simulink model "position_force"  (R2021a)
settings: Solver=FixedStepAuto  StartTime=0.0  StopTime=5  FixedStep=0.001  RelTol=1e-3
values from neighbouring files (symbols this model uses):
  k_fi = 2*eye(3)    [params.m]
  k_fp = 10*eye(3)    [params.m]
  kd = 2*z*w    [params.m]
  kp = w^2    [params.m]
  Md = 0.035*diag([1 1 1])    [params.m]
settings Model: Creator=Sebastiano  LastModifiedBy=antoninoparisi
settings SolverCC: AlgebraicLoopSolver=TrustRegion
settings DebuggingCC: SFMachineParentedDataDiag=warning

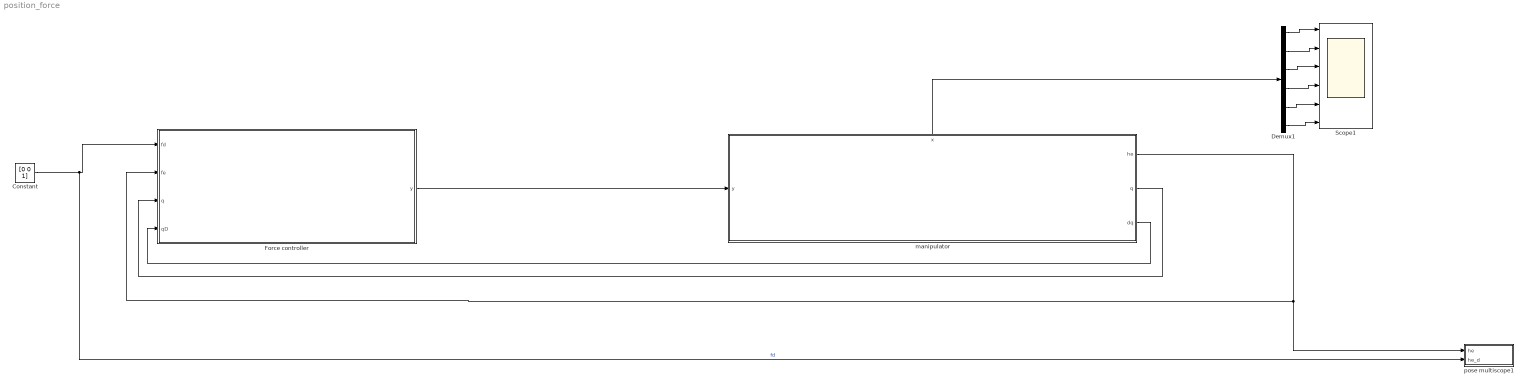
== system position_force ==
  Constant : Constant  Value=[0 0 1]  VectorParams1D=off  SampleTime=0.001
  Demux1 : Demux  Outputs=6
  Force controller : Subsystem
  Scope1 : Scope  NumInputPorts=6
  manipulator : Subsystem
      settings: PortSchema="{\"entries\":[{\"content\":{\"sides\":[{\"content\":{\"connectorIds\":[\"In1\"]},\"type\":\"ConnectorPlacement.EquallySpacedRectSide\",\"uuid\":\"0aa94650-4609-4b6c-9a82-adf30db4dc8c\"},{\"content\":{\"connectorIds\":[\"Out1\",\"Out2\",\"Out3\"],\"side\":\"RIGHT\"},\"type\":\"ConnectorPlacement.EquallySpacedRectSide\",\"uuid\":\"eb872eea-8278-41dd-b116-0828b4bf12ba\"},{\"content\":{\"connectorIds\":[\"Out4\"],\"side\":\"TOP\"},\"type\":\"ConnectorPlacement.EquallySpacedRectSide\",\"uuid\":\"ce640c9d-a400-4b3a-8367-eeadb4eb804b\"}]},\"type\":\"ConnectorPlacement.EquallySpacedConnector\",\"uuid\":\"b8e51044-d9d2-481c-9adb-6cf6a7f6c61e\"}],\"packageUris\":[\"http://schema.mathworks.com/mf0/Connector/R2020b\"],\"version\":\"1.0\"}"
  pose multiscope1 : Subsystem
  wires:
  Constant/1 -> pose multiscope1/2(he_d), Force controller/1(fd)  "fd"
  manipulator/2(q) -> Force controller/3(q)
  manipulator/3(dq) -> Force controller/4(qD)
  manipulator/1(he) -> pose multiscope1/1(he), Force controller/2(fe)
  manipulator/4(x) -> Demux1/1
  Demux1/1 -> Scope1/1
  Demux1/4 -> Scope1/4
  Demux1/5 -> Scope1/5
  Demux1/3 -> Scope1/3
  Demux1/6 -> Scope1/6
  Demux1/2 -> Scope1/2
  Force controller/1(y) -> manipulator/1(y)

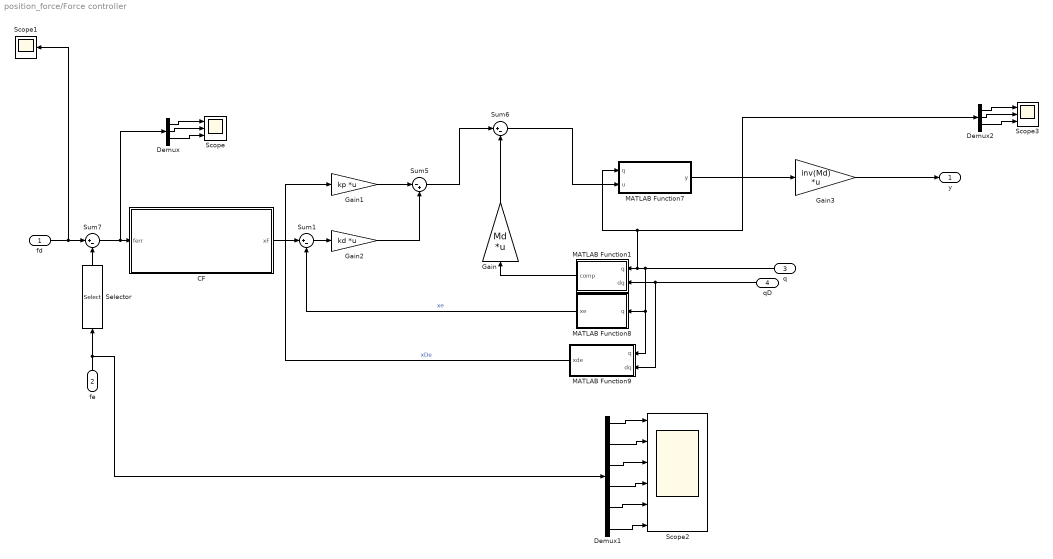
== system position_force/Force controller ==
  fd : Inport
  fe : Inport  Port=2
  q : Inport  Port=3
  qD : Inport  Port=4
  CF : Subsystem
  Demux : Demux  Outputs=3
  Demux1 : Demux  Outputs=6
  Demux2 : Demux  Outputs=3
  Gain : Gain  Gain=Md  Multiplication=Matrix(K*u) (u vector)
  Gain1 : Gain  Gain=kp  Multiplication=Matrix(K*u) (u vector)
  Gain2 : Gain  Gain=kd  Multiplication=Matrix(K*u) (u vector)
  Gain3 : Gain  Gain=inv(Md)  Multiplication=Matrix(K*u) (u vector)
  MATLAB Function1 : MATLAB Function  TreatAsAtomicUnit=on
  MATLAB Function7 : MATLAB Function  TreatAsAtomicUnit=on
  MATLAB Function8 : MATLAB Function  TreatAsAtomicUnit=on
  MATLAB Function9 : MATLAB Function  TreatAsAtomicUnit=on
  Scope : Scope  NumInputPorts=3
  Scope1 : Scope
  Scope2 : Scope  NumInputPorts=6
  Scope3 : Scope  NumInputPorts=3
  Selector : Selector  InputPortWidth=6  IndexOptions=Starting index (dialog)  Indices=1  OutputSizes=3
  Sum1 : Sum  Inputs=|+-
  Sum5 : Sum  Inputs=|-+
  Sum6 : Sum  Inputs=|+-
  Sum7 : Sum  Inputs=|+-
  y : Outport
  wires:
  fd/1 -> Scope1/1, Sum7/1
  Sum1/1 -> Gain2/1
  Sum5/1 -> Sum6/1
  MATLAB Function9/1(xde) -> Gain1/1  "xDe"
  Gain1/1 -> Sum5/1
  MATLAB Function1/1(comp) -> Gain/1
  Sum6/1 -> MATLAB Function7/2(u)
  Gain2/1 -> Sum5/2
  MATLAB Function8/1(xe) -> Sum1/2  "xe"
  Sum7/1 -> Demux/1, CF/1(ferr)
  CF/1(xF) -> Sum1/1
  qD/1 -> MATLAB Function9/2(dq), MATLAB Function1/2(dq)
  q/1 -> Demux2/1, MATLAB Function7/1(q), MATLAB Function1/1(q), MATLAB Function9/1(q), MATLAB Function8/1(q)
  Demux/1 -> Scope/1
  Demux/2 -> Scope/2
  Demux/3 -> Scope/3
  Gain/1 -> Sum6/2
  MATLAB Function7/1(y) -> Gain3/1
  Selector/1 -> Sum7/2
  Demux1/1 -> Scope2/1
  fe/1 -> Demux1/1, Selector/1
  Demux1/2 -> Scope2/2
  Demux1/4 -> Scope2/4
  Demux1/6 -> Scope2/6
  Demux1/5 -> Scope2/5
  Demux1/3 -> Scope2/3
  Demux2/3 -> Scope3/3
  Demux2/2 -> Scope3/2
  Gain3/1 -> y/1
  Demux2/1 -> Scope3/1

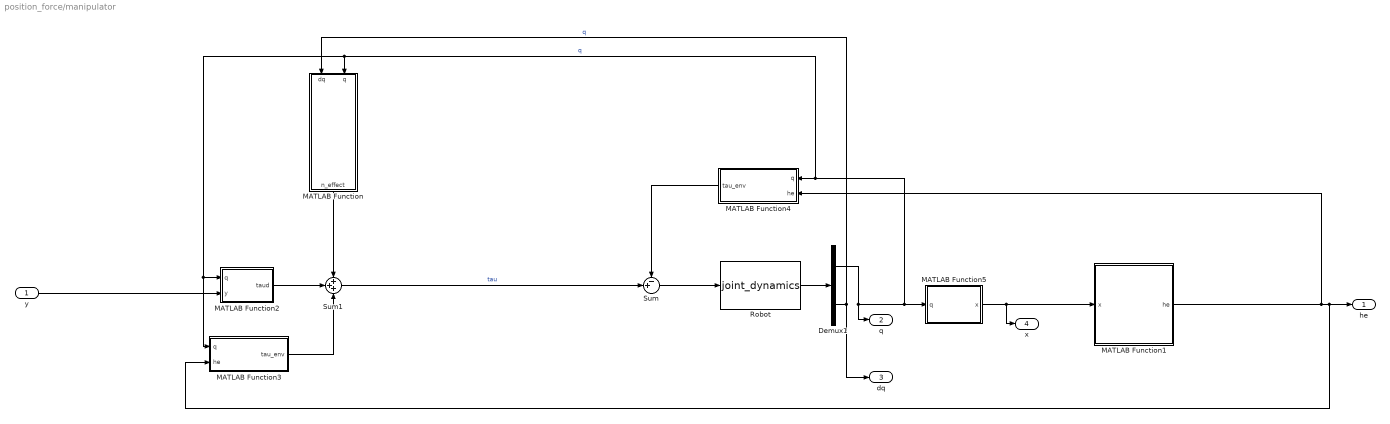
== system position_force/manipulator ==
  y : Inport
  Demux1 : Demux  Outputs=[3, 3]
  MATLAB Function : MATLAB Function  TreatAsAtomicUnit=on
  MATLAB Function1 : MATLAB Function  TreatAsAtomicUnit=on
  MATLAB Function2 : MATLAB Function  TreatAsAtomicUnit=on
  MATLAB Function3 : MATLAB Function  TreatAsAtomicUnit=on
  MATLAB Function4 : MATLAB Function  TreatAsAtomicUnit=on
  MATLAB Function5 : MATLAB Function  TreatAsAtomicUnit=on
  Robot : S-Function  FunctionName=joint_dynamics  Parameters=robot  SFunctionDeploymentMode=off  EnableBusSupport=off
  Sum : Sum  Inputs=-+|
  Sum1 : Sum  Inputs=+++
  he : Outport
  q : Outport  Port=2
  dq : Outport  Port=3
  x : Outport  Port=4
  wires:
  Sum/1 -> Robot/1
  Robot/1 -> Demux1/1
  MATLAB Function4/1(tau_env) -> Sum/1
  MATLAB Function5/1(x) -> x/1, MATLAB Function1/1(x)
  MATLAB Function1/1(he) -> MATLAB Function4/2(he), MATLAB Function3/2(he), he/1
  Demux1/1 -> MATLAB Function5/1(q), MATLAB Function/2(q), MATLAB Function3/1(q), MATLAB Function2/1(q), MATLAB Function4/1(q), q/1  "q"
  y/1 -> MATLAB Function2/2(y)
  MATLAB Function/1(n_effect) -> Sum1/1
  Sum1/1 -> Sum/2  "tau"
  MATLAB Function3/1(tau_env) -> Sum1/3
  MATLAB Function2/1(taud) -> Sum1/2
  Demux1/2 -> dq/1, MATLAB Function/1(dq)  "q"

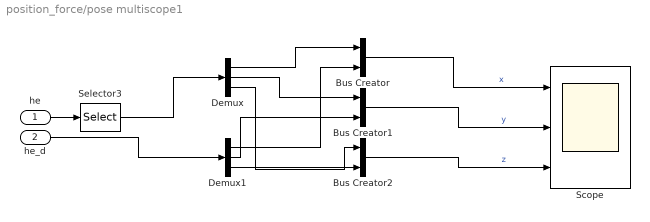
== system position_force/pose multiscope1 ==
  he : Inport
  he_d : Inport  Port=2
  Bus Creator : BusCreator  Inputs=2
  Bus Creator1 : BusCreator  Inputs=2
  Bus Creator2 : BusCreator  Inputs=2
  Demux : Demux  Outputs=3
  Demux1 : Demux  Outputs=3
  Scope : Scope  NumInputPorts=3
  Selector3 : Selector  InputPortWidth=6  IndexOptions=Starting index (dialog)  Indices=1  OutputSizes=3
  wires:
  he_d/1 -> Demux1/1
  he/1 -> Selector3/1
  Selector3/1 -> Demux/1
  Demux/1 -> Bus Creator/1
  Demux1/1 -> Bus Creator/2
  Demux/2 -> Bus Creator1/1
  Demux/3 -> Bus Creator2/1
  Demux1/2 -> Bus Creator1/2
  Demux1/3 -> Bus Creator2/2
  Bus Creator/1 -> Scope/1  "x"
  Bus Creator1/1 -> Scope/2  "y"
  Bus Creator2/1 -> Scope/3  "z"

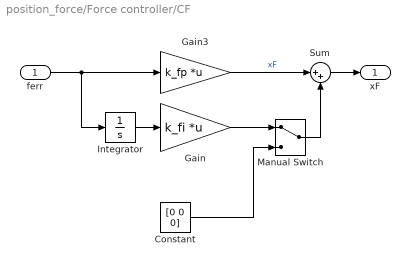
== system position_force/Force controller/CF ==
  ferr : Inport
  Constant : Constant  Value=[0 0 0]
  Gain : Gain  Gain=k_fi  Multiplication=Matrix(K*u) (u vector)
  Gain3 : Gain  Gain=k_fp  Multiplication=Matrix(K*u) (u vector)
  Integrator : Integrator
  Manual Switch : ManualSwitch
  Sum : Sum  Inputs=|++
  xF : Outport
  wires:
  ferr/1 -> Integrator/1, Gain3/1
  Gain3/1 -> Sum/1  "xF"
  Sum/1 -> xF/1
  Gain/1 -> Manual Switch/1
  Manual Switch/1 -> Sum/2
  Integrator/1 -> Gain/1
  Constant/1 -> Manual Switch/2

== matlab function position_force/Force controller/MATLAB Function7 ==
  data: q input; u input; y output
function y = Jpinv(q, u)

J = jacobian(q);
Jp = J(1:3,:);
y =  pinv(Jp) * u;

== matlab function position_force/Force controller/MATLAB Function1 ==
  data: q input; comp output; dq input
function comp = JpD(q, dq)

   
Jpd = jacobian_dot(q,dq);

Jpd = Jpd(1:3,:);

comp = Jpd*dq;

== matlab function position_force/Force controller/MATLAB Function8 ==
  data: q input; xe output
function xe = Kp(q)

t1 = q(1);
d1 = q(2);
t2 = q(3);


a1 = 0.15;
a2 = 0.4;
a3 = 0.3;
a4 = 0.16;


K = [[cos(t1)*cos(t2), -cos(t1)*sin(t2), -sin(t1),      a2*cos(t1) + a4*cos(t1)*cos(t2)]
    [        sin(t2),          cos(t2),        0,                 a4*sin(t2) - d1 - a3]
    [cos(t2)*sin(t1), -sin(t1)*sin(t2),  cos(t1), a1 + a2*sin(t1) + a4*cos(t2)*sin(t1)]
    [              0,                0,        0,                                    1]];

xe = K(1:3, 4);

== matlab function position_force/Force controller/MATLAB Function9 ==
  data: q input; xde output; dq input
function xde = Jp(q, dq)

J = jacobian(q);
Jp = J(1:3,:);
xde = Jp * dq;

== matlab function position_force/manipulator/MATLAB Function ==
  data: dq input; q input; n_effect output
function n_effect = n(dq, q)

n_effect = C_Lagrangian(q, dq)*dq + G_Lagrangian(q);

== matlab function position_force/manipulator/MATLAB Function1 ==
  data: x input; he output
function he = environment(x)

% environment params
K = diag([2 2 2 0.1 0.1 0.1])*10;    % stiffness
wall = 0.16; % constraint position w.r.t. frame 0 (it's y=-0.5 w.r.t. base frame)

if abs(x(3)) >= wall  % check is done in frame 0
    % touching the environment! constrained motion
    % set up the rest position frame
    % (basically, same orientation as ee but position is the contact point at the wall)
    xr = x;
    xr(3) = wall;
    % calculate the forces
    dx_re = x - xr;
    he = K * dx_re;
else
    % free motion
    he = zeros(6,1);
end

he = reshape(he,[6 1]);

== matlab function position_force/manipulator/MATLAB Function2 ==
  data: q input; taud output; y input
function taud = B(q, y)

taud = B_Lagrangian(q)*y;

== matlab function position_force/manipulator/MATLAB Function3 ==
  data: q input; he input; tau_env output
function tau_env = J(q, he)

tau_env = jacobian(q)' * he;

== matlab function position_force/manipulator/MATLAB Function4 ==
  data: q input; he input; tau_env output
function tau_env = J(q, he)

tau_env = jacobian(q)' * he;

== matlab function position_force/manipulator/MATLAB Function5 ==
  data: q input; x output
function x = K(q)

t1 = q(1);
d1 = q(2);
t2 = q(3);


a1 = 0.15;
a2 = 0.4;
a3 = 0.3;
a4 = 0.16;


% wrt frame 0
K = [[cos(t1)*cos(t2), -cos(t1)*sin(t2), -sin(t1),      a2*cos(t1) + a4*cos(t1)*cos(t2)]
    [        sin(t2),          cos(t2),        0,                 a4*sin(t2) - d1 - a3]
    [cos(t2)*sin(t1), -sin(t1)*sin(t2),  cos(t1), a1 + a2*sin(t1) + a4*cos(t2)*sin(t1)]
    [              0,                0,        0,                                    1]];

pos = K(1:3, 4);
ori = rotm2eul(K(1:3,1:3), 'ZYZ')';

x = [pos; ori];
